simulink model "Lab07A"  (R2021a)
settings: Solver=VariableStepAuto  StartTime=0.0  StopTime=10.0  RelTol=1e-3
undefined symbols (not defined in the file): DiscIntNeverNeededParam
settings Model: Creator=shirs  LastModifiedBy=shirs

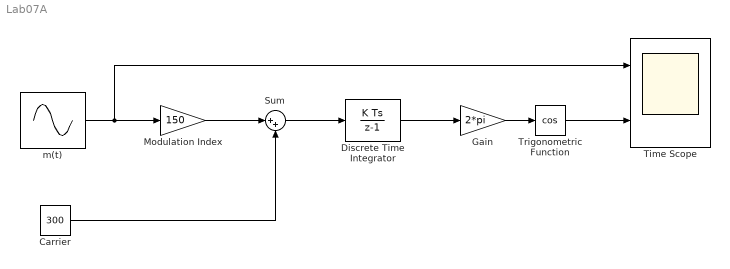
== system Lab07A ==
  Carrier : Constant  Value=300
  Discrete Time Integrator : DiscreteIntegrator  SampleTime=1/98000  ICPrevOutput=DiscIntNeverNeededParam  ICPrevScaledInput=DiscIntNeverNeededParam
  Gain : Gain  Gain=2*pi
  Modulation Index : Gain  Gain=150
  Sum : Sum  Inputs=|++
  Time Scope : Scope  NumInputPorts=2
  Trigonometric Function : Trigonometry  Operator=cos
  m(t) : Sin  Frequency=10  Phase=90  SampleTime=1/98000
  wires:
  Carrier/1 -> Sum/2
  m(t)/1 -> Time Scope/1, Modulation Index/1
  Modulation Index/1 -> Sum/1
  Sum/1 -> Discrete Time Integrator/1
  Discrete Time Integrator/1 -> Gain/1
  Gain/1 -> Trigonometric Function/1
  Trigonometric Function/1 -> Time Scope/2
